simulink model "GasTurbine_Dyn_Template"  (R2015a)
settings: Solver=ode4  StartTime=0.0  StopTime=MWS.in.SimTime  FixedStep=MWS.Solve.T  RelTol=1e-3
values from neighbouring files (symbols this model uses):
  MWS = setup_Inlet(MWS)    [GasTurbine_Dyn_setup_everything.m]
libraries: Lib_Solve_ModelSource_TMATS x2, Lib_Cntrl_FirstOrderSensor_TMATS x1, Lib_Solve_IterNRSolverJC_TMATS x1, Lib_Solve_OuterLoopIntegrator_TMATS x1
CloseFcn:
  | run(strcat(MWS.top_level, filesep,'GasTurbine_Dyn_Example_cleanup'))
settings Model: Creator=jwchapm2  LastModifiedBy=jwchapm2
settings DataIOCC: SignalLoggingName=SimulationOutput
settings OptimizationCC: BlockReduction=off  InlineParams=on  BufferReuse=off  ExpressionDepthLimit=2147483647
settings DebuggingCC: UnderspecifiedInitializationDetection=Classic  MergeDetectMultiDrivingBlocksExec=none  SolverPrmCheckMsg=warning  StateNameClashWarn=warning

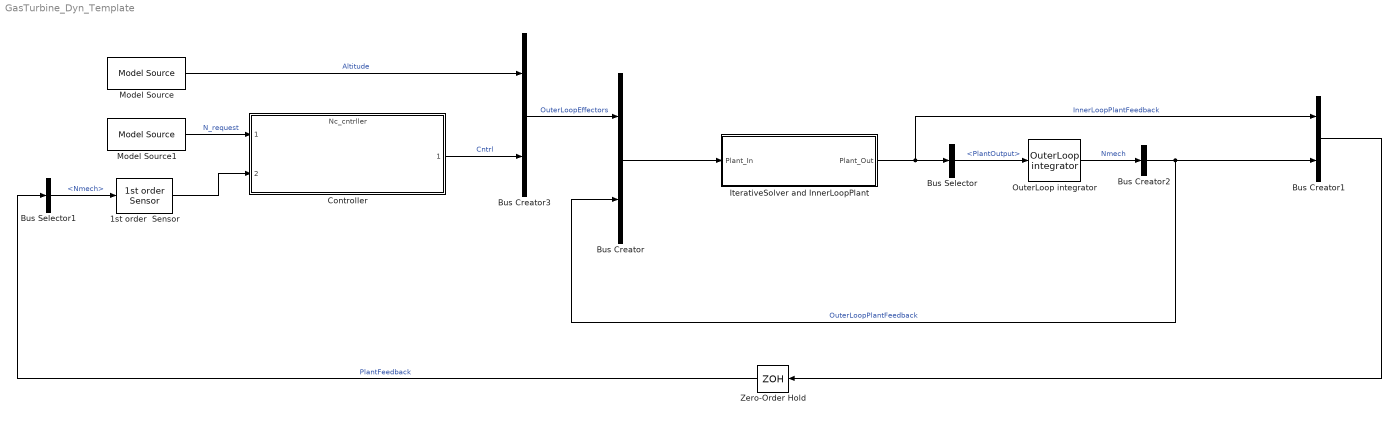
== system GasTurbine_Dyn_Template ==
  1st order  Sensor : Lib_Cntrl_FirstOrderSensor_TMATS/1st order  Sensor  IC_M=MWS.Solve.N_IC  Sen_Max_M=20000  Sen_Min_M=0  Gain_M=1  Tau_M=0.05  GN_EN_M=off  GN_NST_M=MWS.Solve.T  GN_C_M=1  GN_MinNoise_M=0.3  F_Gain_M=1  F_Drift_M=0
  Bus Creator : BusCreator  Inputs=2
  Bus Creator1 : BusCreator  Inputs=2
  Bus Creator2 : BusCreator  Inputs=1
  Bus Creator3 : BusCreator  Inputs=2
  Bus Selector : BusSelector  OutputSignals=PlantOutput
  Bus Selector1 : BusSelector  OutputSignals=OuterLoopPlantFeedback.Nmech
  Controller : ModelReference  ModelNameDialog=Nc_cntrller  SimulationMode=Normal  ModelReferenceVersion=1.29  CopyOfModelName=Nc_cntrller  DefaultDataLogging=on
      settings: AttributesFormatString=%<ActiveVariant>
  IterativeSolver and InnerLoopPlant : Subsystem
  Model Source : Lib_Solve_ModelSource_TMATS/Model Source  T_vec_M=MWS.in.t_vec  input_array_M=MWS.in.Alt
  Model Source1 : Lib_Solve_ModelSource_TMATS/Model Source  T_vec_M=MWS.in.t_vec  input_array_M=MWS.in.Ndmd
  OuterLoop integrator : Lib_Solve_OuterLoopIntegrator_TMATS/OuterLoop integrator  OL_IC_M=MWS.Solve.N_IC
  Zero-Order Hold : ZeroOrderHold  SampleTime=MWS.Solve.T
  wires:
  Zero-Order Hold/1 -> Bus Selector1/1  "PlantFeedback"
  Bus Creator/1 -> IterativeSolver and InnerLoopPlant/1(Plant_In)
  IterativeSolver and InnerLoopPlant/1(Plant_Out) -> Bus Selector/1, Bus Creator1/1  "InnerLoopPlantFeedback"
  Bus Selector/1 -> OuterLoop integrator/1  "<PlantOutput>"
  Bus Creator2/1 -> Bus Creator/2, Bus Creator1/2  "OuterLoopPlantFeedback"
  Bus Creator3/1 -> Bus Creator/1  "OuterLoopEffectors"
  Bus Creator1/1 -> Zero-Order Hold/1
  OuterLoop integrator/1 -> Bus Creator2/1  "Nmech"
  Bus Selector1/1 -> 1st order  Sensor/1  "<Nmech>"
  Controller/1 -> Bus Creator3/2  "Cntrl"
  Model Source1/1 -> Controller/1  "N_request"
  1st order  Sensor/1 -> Controller/2
  Model Source/1 -> Bus Creator3/1  "Altitude"

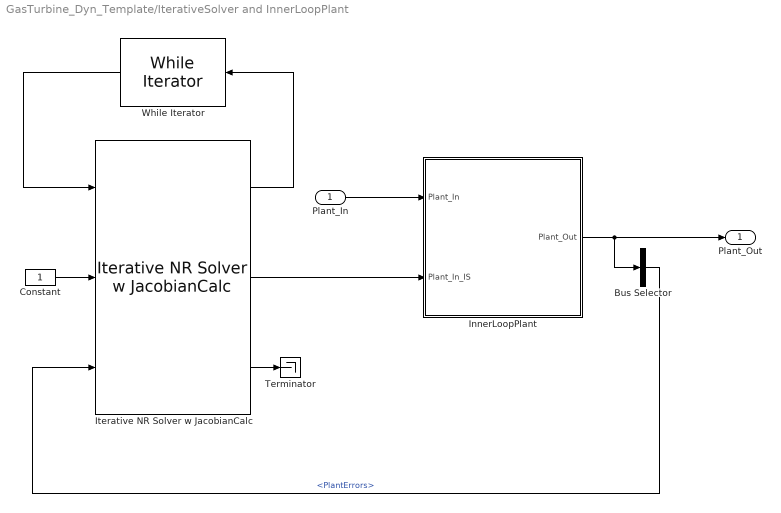
== system GasTurbine_Dyn_Template/IterativeSolver and InnerLoopPlant ==
  Plant_In : Inport  OutDataTypeStr=Bus: PlantInputs
  Bus Selector : BusSelector  OutputSignals=PlantErrors
  Constant : Constant
  InnerLoopPlant : Subsystem
  Iterative NR Solver w JacobianCalc : Lib_Solve_IterNRSolverJC_TMATS/Iterative NR Solver w JacobianCalc  SJac_Per_M=MWS.Solve.J_Calc_Per  SNR_IC_M=MWS.Solve.NR_IC  SNR_DX_M=MWS.Solve.NR_dx  SNR_Mx_M=100000  SNR_Mn_M=0.0001  SJacobianAttempts_M=MWS.Solve.NR_Jac_Re  Cond_Limits_M=0.01
  Terminator : Terminator
  While Iterator : WhileIterator  MaxIters=MWS.Solve.Max_Iter  WhileBlockType=do-while  ShowIterationPort=on
  Plant_Out : Outport
  wires:
  Plant_In/1 -> InnerLoopPlant/1(Plant_In)
  Bus Selector/1 -> Iterative NR Solver w JacobianCalc/3  "<PlantErrors>"
  While Iterator/1 -> Iterative NR Solver w JacobianCalc/1
  InnerLoopPlant/1(Plant_Out) -> Bus Selector/1, Plant_Out/1
  Iterative NR Solver w JacobianCalc/2 -> InnerLoopPlant/2(Plant_In_IS)
  Iterative NR Solver w JacobianCalc/1 -> While Iterator/1
  Iterative NR Solver w JacobianCalc/3 -> Terminator/1
  Constant/1 -> Iterative NR Solver w JacobianCalc/2

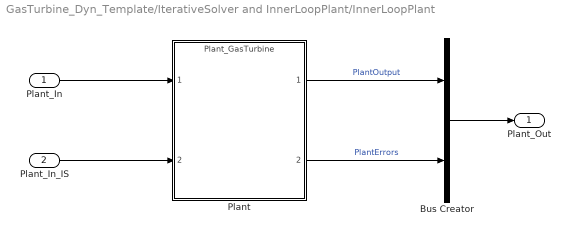
== system GasTurbine_Dyn_Template/IterativeSolver and InnerLoopPlant/InnerLoopPlant ==
  Plant_In : Inport  OutDataTypeStr=Bus: PlantInputs
  Plant_In_IS : Inport  Port=2
  Bus Creator : BusCreator  Inputs=2
  Plant : ModelReference  ModelNameDialog=Plant_GasTurbine  SimulationMode=Normal  ModelReferenceVersion=1.119  CopyOfModelName=Plant_GasTurbine  DefaultDataLogging=on
      settings: AttributesFormatString=%<ActiveVariant>
  Plant_Out : Outport
  wires:
  Plant/1 -> Bus Creator/1  "PlantOutput"
  Plant/2 -> Bus Creator/2  "PlantErrors"
  Plant_In/1 -> Plant/1
  Plant_In_IS/1 -> Plant/2
  Bus Creator/1 -> Plant_Out/1
